simulink model "ex3"  (R2015a)
settings: Solver=ode4  StartTime=0.0  StopTime=20.0  FixedStep=0.01  RelTol=1e-3
values from neighbouring files (symbols this model uses):
  A = [0 0 0; 1 0 -1; 0 1 2]    [ex1.m]
  B = [0 -1; 1 0; 0 1]    [ex1.m]
  C = [1 0 1]    [ex1.m]
  F = F0 + g * f_T    [ex1.m]
  G = eye(m)    [ex1.m]
settings Model: Creator=Cazan Bogdan  LastModifiedBy=andre

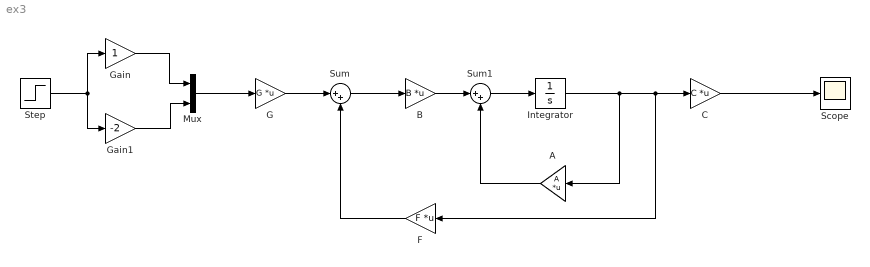
== system ex3 ==
  A : Gain  Gain=A  Multiplication=Matrix(K*u)
  B : Gain  Gain=B  Multiplication=Matrix(K*u)
  C : Gain  Gain=C  Multiplication=Matrix(K*u)
  F : Gain  Gain=F  Multiplication=Matrix(K*u)
  G : Gain  Gain=G  Multiplication=Matrix(K*u)
  Gain : Gain
  Gain1 : Gain  Gain=-2
  Integrator : Integrator
  Mux : Mux  Inputs=2
  Scope : Scope
      settings: TimeRange=20  YMin=-5000000000  YMax=3000000000
  Step : Step  SampleTime=0
  Sum : Sum  Inputs=|++
  Sum1 : Sum  Inputs=|++
  wires:
  Step/1 -> Gain1/1, Gain/1
  Gain/1 -> Mux/1
  Gain1/1 -> Mux/2
  G/1 -> Sum/1
  Sum/1 -> B/1
  F/1 -> Sum/2
  C/1 -> Scope/1
  Mux/1 -> G/1
  B/1 -> Sum1/1
  Sum1/1 -> Integrator/1
  A/1 -> Sum1/2
  Integrator/1 -> A/1, F/1, C/1
